simulink model "msv_sim_updated"  (R2021b)
settings: Solver=VariableStepAuto  StartTime=0.0  StopTime=100  RelTol=1e-3
settings Model: Creator=ishaa  LastModifiedBy=ishaa

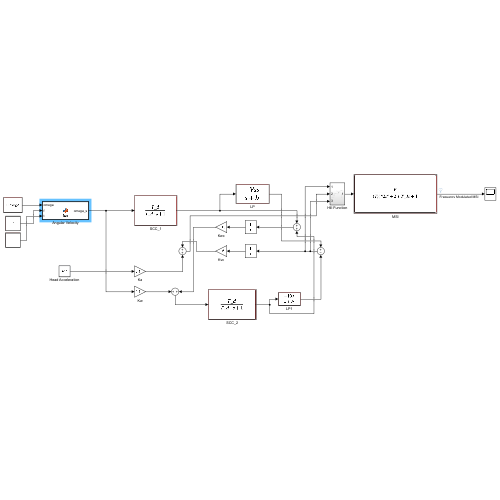
[thumbnail: Simulink's stored preview of the top-level diagram]
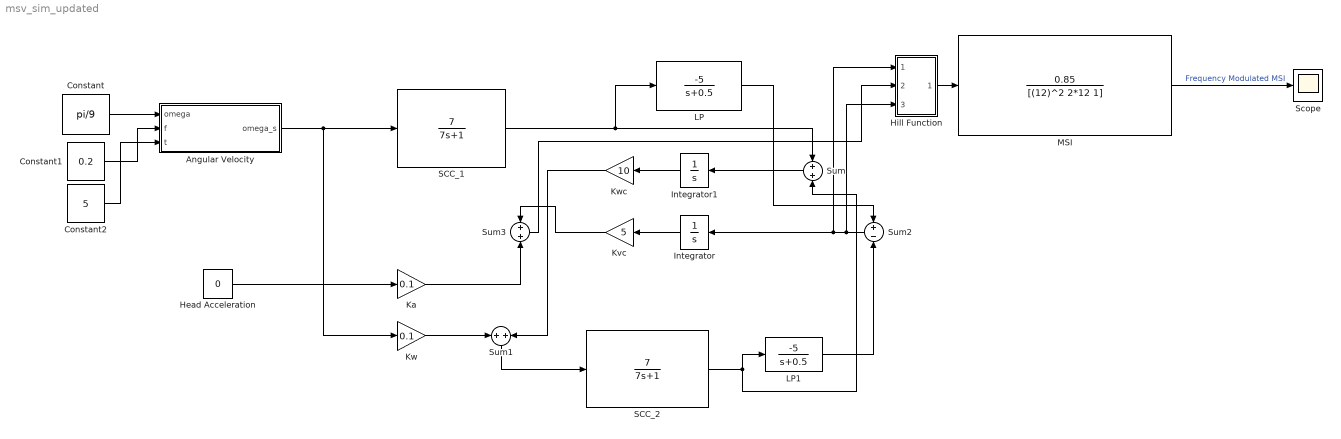
== system msv_sim_updated ==
  Angular Velocity : MATLAB Function  TreatAsAtomicUnit=on
  Constant : Constant  Value=pi/9
      mask Display: image('C:\Users\ishaa\Downloads\1.PNG'); % Use "Edit Image" on toolstrip to change.
  Constant1 : Constant  Value=0.2
      mask Display: image('C:\Users\ishaa\Downloads\2.PNG'); % Use "Edit Image" on toolstrip to change.
  Constant2 : Constant  Value=5
      mask Display: image('C:\Users\ishaa\Downloads\3.PNG'); % Use "Edit Image" on toolstrip to change.
  Head Acceleration : Constant  Value=0
      mask Display: image('C:\Users\ishaa\Downloads\Screenshot 2022-04-24 224719.png'); % Use "Edit Image" on toolstrip to change.
  Hill Function : Subsystem
  Integrator : Integrator
  Integrator1 : Integrator
  Ka : Gain  Gain=0.1
  Kvc : Gain  Gain=5
  Kw : Gain  Gain=0.1
  Kwc : Gain  Gain=10
  LP : TransferFcn  Numerator=[-5]  Denominator=[1 0.5]
      mask Display: image('C:\Users\ishaa\Downloads\new.PNG'); % Use "Edit Image" on toolstrip to change.
  LP1 : TransferFcn  Numerator=[-5]  Denominator=[1 0.5]
      mask Display: image('C:\Users\ishaa\Downloads\new.PNG'); % Use "Edit Image" on toolstrip to change.
  MSI : TransferFcn  Numerator=[0.85]  Denominator=[(12)^2 2*12 1]
      mask Display: image('C:\Users\ishaa\Downloads\5.PNG'); % Use "Edit Image" on toolstrip to change.
  SCC_1 : TransferFcn  Numerator=[7]  Denominator=[7 1]
      mask Display: image('C:\Users\ishaa\Downloads\4.PNG'); % Use "Edit Image" on toolstrip to change.
  SCC_2 : TransferFcn  Numerator=[7]  Denominator=[7 1]
      mask Display: image('C:\Users\ishaa\Downloads\4.PNG'); % Use "Edit Image" on toolstrip to change.
  Scope : Scope
  Sum : Sum
  Sum1 : Sum
  Sum2 : Sum  Inputs=+-
  Sum3 : Sum
  wires:
  SCC_1/1 -> LP/1, Sum/1
  Sum/1 -> Integrator1/1
  Sum1/1 -> SCC_2/1
  SCC_2/1 -> LP1/1, Sum/2
  LP/1 -> Sum2/1
  Sum2/1 -> Hill Function/1(In1), Integrator/1, Hill Function/3(In2)
  Integrator/1 -> Kvc/1
  Integrator1/1 -> Kwc/1
  Angular Velocity/1(omega_s) -> Kw/1, SCC_1/1
  Head Acceleration/1 -> Ka/1
  LP1/1 -> Sum2/2
  Kvc/1 -> Sum3/1
  Ka/1 -> Sum3/2
  Kw/1 -> Sum1/1
  Kwc/1 -> Sum1/2
  MSI/1 -> Scope/1  "Frequency Modulated MSI"
  Hill Function/1(Out1) -> MSI/1
  Constant2/1 -> Angular Velocity/3(t)
  Constant1/1 -> Angular Velocity/2(f)
  Constant/1 -> Angular Velocity/1(omega)
  Sum3/1 -> Hill Function/2(In3)

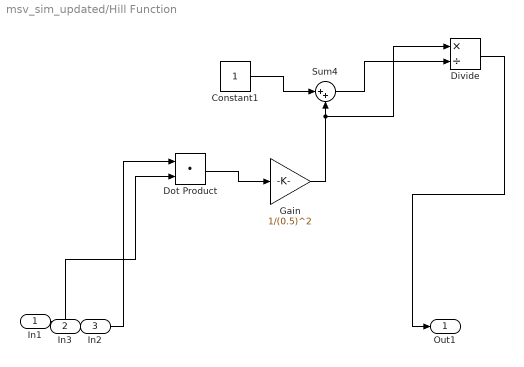
== system msv_sim_updated/Hill Function ==
  In1 : Inport
  In3 : Inport  Port=2
  In2 : Inport  Port=3
  Constant1 : Constant
  Divide : Product  Inputs=*/
  Dot Product : DotProduct  InputSameDT=on  OutDataTypeStr=Inherit: Inherit via internal rule
  Gain : Gain  Gain=1/(0.5)^2
  Sum4 : Sum  Inputs=|++
  Out1 : Outport
  wires:
  Divide/1 -> Out1/1
  Gain/1 -> Divide/1, Sum4/2
  Constant1/1 -> Sum4/1
  In1/1 -> Dot Product/2
  Dot Product/1 -> Gain/1
  In2/1 -> Dot Product/1
  Sum4/1 -> Divide/2

== matlab function msv_sim_updated/Angular Velocity ==
  data: omega input; omega_s output; f input; t input
function omega_s = fcn(omega, f, t)
omega_s = (sqrt(2)*omega*(sin(2*pi))*f*t);
end
